simulink model "rgpio_test"  (Simulink 7.6)
settings: Solver=FixedStepDiscrete  StartTime=0.0  StopTime=Inf  RelTol=1e-3
libraries: rpi_blkst x1
settings Model: Creator=jacques  LastModifiedBy=jacques
settings OptimizationCC: OptimizeModelRefInitCode=on  LifeSpan=1
settings HardwareCC: ProdLargestAtomicInteger=Long  ProdLargestAtomicFloat=Double  ProdEndianess=LittleEndian  ProdHWDeviceType=ARM Compatible->ARM 11
settings RTWCC: SystemTargetFile=ert_rpi.tlc  TemplateMakefile=ert_rpi.tmf  PostCodeGenCommand=postGenFunc(buildInfo)  Description=RTW Embedded Coder RPI target  ProcessScript=ert_rpi_make_rtw_hook
settings CodeAppCC: IgnoreCustomStorageClasses=off
settings STFCustomTargetCC: ModelReferenceCompliant=off  CombineOutputUpdateFcns=on  ERTCustomFileBanners=on  SupportNonInlinedSFcns=off  SystemTargetFile=ert_rpi.tlc
settings ERTTargetCC: MultiwordLength=2048  ModelReferenceCompliant=off  ParMdlRefBuildCompliant=off  CompOptLevelCompliant=off  ERTFirstTimeCompliant=off  SupportContinuousTime=on  ModelStepFunctionPrototypeControlCompliant=off  CPPClassGenCompliant=off  ExtMode=on  ExtModeMexArgs='130.79.72.217'  InlinedParameterPlacement=NonHierarchical  ERTCustomFileTemplate=ert_rpi_file_process.tlc  ConvertIfToSwitch=off

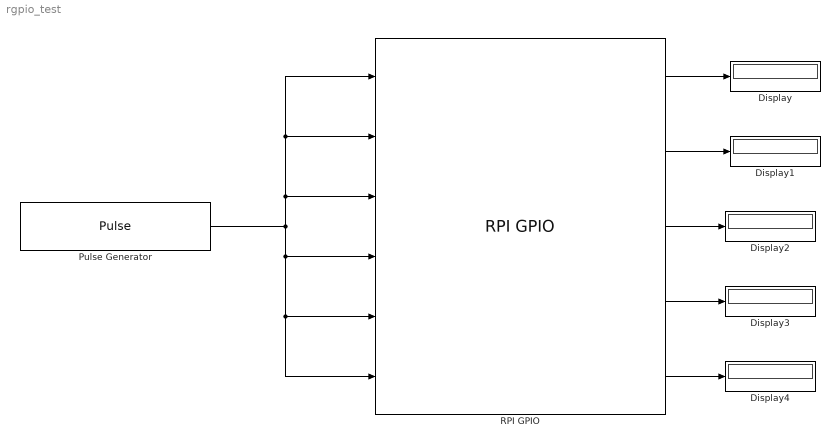
== system rgpio_test ==
  Display{,1..4} (5 alike) : Display
  Pulse Generator : DiscretePulseGenerator  Period=1000  PulseWidth=500  SampleTime=0.001
  RPI GPIO : rpi_blkst/RPI GPIO  SystemSampleTime=-1  rpi_mask_Ts=0.001
  wires:
  Pulse Generator/1 -> RPI GPIO/1, RPI GPIO/2, RPI GPIO/3, RPI GPIO/4, RPI GPIO/5, RPI GPIO/6
  RPI GPIO/1 -> Display/1
  RPI GPIO/2 -> Display1/1
  RPI GPIO/3 -> Display2/1
  RPI GPIO/4 -> Display3/1
  RPI GPIO/5 -> Display4/1
